simulink model "ATOM_simple_planning_simulator"  (R2026a)
settings: Solver=ode4  StopTime=50  FixedStep=0.01
StopFcn:
  | if exist('costmap_active','var') && ...
  |    exist('vehicle','var') && ...
  |    exist('parking_path','var') && ...
  |    ~isempty(parking_path)
  | 
  |     plotPlan(costmap_active, vehicle, parking_path);
  | else
  |     warning('No valid parking path is available for plotting.');
  | end
model workspace (MAT data in the model file):
  vehicle : object (value not decoded)
symbols that are objects in the model workspace (value not decoded): vehicle
undefined symbols (not defined in the file or in its folder): delta_f_LUT, gain4WS_LUT, k_ref_LUT, kappa_gain_BP, Ki, Kp, lateral, longitudinal, planning_validator, rr_gain_BP, rr_LUT, stanley, velocity_smoother
libraries: slpidlib x1, simulink x1
(part 6 of 7)

== matlab function ATOM_simple_planning_simulator/Subsystem/parkingNMPC ==
  settings: updateMethod=DISCRETE  sampleTime=0.04
  data: tx input; path_length output; ty input; tqz input; tqw input; tdf input; tdr input; tvx input; tax input; max_q output; X input; Y input; s_now output; ey_now output; qz input; qw input; vx input; ax_meas input; df input; dr input; x_now output; veh input; longitudinal_mode output; df_cmd output; dr_cmd output; nmpc_info output; segment_done output; segment_changed input; endpoint_error output; a_cmd_previous input; costmap input
function [path_length, max_q, s_now, ey_now, x_now, ...
    longitudinal_mode, df_cmd, dr_cmd, nmpc_info, ...
    segment_done, endpoint_error] = parkingNMPC( ...
    tx,ty,tqz,tqw,tdf,tdr,tvx,tax, ...
    X,Y,qz,qw,vx,ax_meas,df,dr,veh, ...
    segment_changed,a_cmd_previous,costmap)
persistent ref s_prev U_prev buf aBuf terminal_creep_steps

N  = 15;
nd = 6;

% Build the reference during the first execution.
if isempty(ref)
    ref = buildRef(tx,ty,tqz,tqw,tdf,tdr,tvx,tax);
end

if isempty(s_prev)
    s_prev = 0;
end

if isempty(U_prev)
    U_prev = repmat([df, dr], N, 1);
end

if isempty(buf)
    % Initialize the delayed-command history from the measured wheel angles.
    buf = repmat([df, dr], nd, 1);
end

% History of acceleration commands already sent to the vehicle.
% Three samples are retained because the acceleration delay is 0.10 s,
% equivalent to 2.5 controller intervals at Ts = 0.04 s.
if isempty(aBuf)
    aBuf = repmat(a_cmd_previous,3,1);
else
    aBuf = [aBuf(2:end); a_cmd_previous];
end

if isempty(terminal_creep_steps)
    terminal_creep_steps = 0.0;
end

% Rebuild the reference once when the segment changes.
if logical(segment_changed)
    ref = buildRef(tx,ty,tqz,tqw,tdf,tdr,tvx,tax);
    s_prev = 0;
    U_prev = repmat([df,dr],N,1);
    terminal_creep_steps = 0.0;
end
path_length = ref.s(end); max_q = max(ref.q);
[s_new, ey_now] = whereOnPath(ref, X, Y, s_prev);
s_now  = min(max(s_new, s_prev), s_prev + 0.5);   % never backwards, never a big jump forward
s_prev = s_now;

% --- the state of the car right now ---
psi   = 2*atan2(qz, qw);
x_now = [X; Y; psi; vx; df; dr; ax_meas]; %state of the nmpc controller
P     = carNumbers(veh);
M = mapNumbers(costmap);

% Remaining path distance used by the maneuver supervisor.
d_left = max(ref.s(end) - s_now, 0);

% The segment is complete only after reaching its end and stopping.
% Actual distance from the vehicle's rear axle to the segment endpoint.
endpoint_distance = hypot( ...
    X - ref.X(end), ...
    Y - ref.Y(end));

% Heading error relative to the segment endpoint, wrapped to [-pi, pi].
heading_difference = psi - ref.psi(end);

endpoint_heading_error = atan2( ...
    sin(heading_difference), ...
    cos(heading_difference));

% ---------------- Segment arrival and stop supervision ----------------
%
% Precise tolerance:
% Used to evaluate the final tracking quality.
%
% Arrival tolerance:
% Used to decide whether the stopped vehicle may proceed to the next
% forward/reverse segment.

end_distance_tolerance = 0.05;       % [m]
end_heading_tolerance  = 2*pi/180;   % [rad]

arrive_distance_tolerance = 0.20;       % [m]
arrive_heading_tolerance  = 5*pi/180;   % [rad]

stop_speed_tolerance = 0.02;         % [m/s]

% Because s_now is not allowed to decrease, end_reached remains true
% after the vehicle reaches the final path progress.
end_reached = ...
    d_left <= 0.02;

% High-accuracy endpoint condition.
pose_acceptable = ...
    (endpoint_distance <= end_distance_tolerance) && ...
    (abs(endpoint_heading_error) <= end_heading_tolerance);

% Practical condition for authorizing the next gear segment.
pose_arrived = ...
    (endpoint_distance <= arrive_distance_tolerance) && ...
    (abs(endpoint_heading_error) <= arrive_heading_tolerance);

% The vehicle must be nearly stationary before changing segments.
stopped = ...
    abs(vx) <= stop_speed_tolerance;

% Advance to the next segment only after reaching the endpoint progress,
% stopping, and satisfying the practical arrival tolerance.
segment_done = ...
    end_reached && ...
    stopped && ...
    pose_arrived;

% If the vehicle stops outside the arrival tolerance, keep the current
% segment active and report the failure through the controller status.
arrival_failed = ...
    end_reached && ...
    stopped && ...
    ~pose_arrived;

% Permanent endpoint diagnostics:
%   element 1: position error [m]
%   element 2: signed heading error [deg]
endpoint_error = [ ...
    endpoint_distance; ...
    endpoint_heading_error*180/pi];

% Longitudinal modes:
%   0 = follow the planned velocity profile
%   2 = stop
%
% Once endpoint progress is reached, stop mode remains active.
% Terminal creep mode is deliberately removed.
longitudinal_mode = 0.0;

if end_reached
    longitudinal_mode = 2.0;
end

% --- steering ---
use_nmpc = true;      % false = D1 baseline (follow the plan blindly)
w = [10 10 1 0.1];     % weights: side error, heading error, wheel error, command jumps

if use_nmpc
    x0   = x_now;                                          % start from the real car
    cost = @(u) score( ...
        reshape(u,N,2), ...
        x0, ...
        s_now, ...
        buf, ...
        aBuf, ...
        ref, ...
        P, ...
        w, ...
        longitudinal_mode);

    nonlinear_constraint = @(u) collisionConstraints( ...
        u, ...
        x0, ...
        s_now, ...
        buf, ...
        aBuf, ...
        ref, ...
        P, ...
        M, ...
        longitudinal_mode);

    lb   = -P.steerMax*ones(2*N,1);                        % wheel limits
    ub   =  P.steerMax*ones(2*N,1);
    % Shared tolerance for the optimizer and the independent collision check.
    collision_tolerance = 1e-6;
    
    opts = optimoptions('fmincon', ...
        'Algorithm', 'sqp', ...
        'Display', 'none', ...
        'MaxIterations', 30, ...
        'ConstraintTolerance', collision_tolerance);
    solve_start = tic;
    
    % Optimize the front and rear steering commands.
    % Steering-angle limits are hard constraints.
    % Command changes are discouraged by the dU term in the cost function.
    [u, J_best, flag, solver_output] = fmincon( ...
        cost, U_prev(:), ...
        [], [], [], [], ...
        lb, ub, ...
        nonlinear_constraint, opts);
    
    solve_time = toc(solve_start);
    % Check whether the returned cost and commands are finite.
    finite_solution = ...
        isfinite(J_best) && ...
        all(isfinite(u));

    % Small tolerance for numerical round-off at the steering limits.
    bound_tolerance = 1e-9;

    % Check whether all optimized commands respect their bounds.
    inside_bounds = ...
        all(u >= lb - bound_tolerance) && ...
        all(u <= ub + bound_tolerance);

    % Verify the nonlinear collision constraints independently after
    % fmincon returns its candidate solution.
    collision_feasible = false;

    % Do not evaluate geometric constraints using nonfinite commands or
    % a candidate already declared invalid by the solver.
    if finite_solution && flag >= 0

        [candidate_collision_constraints,~] = ...
            collisionConstraints( ...
            u, ...
            x0, ...
            s_now, ...
            buf, ...
            aBuf, ...
            ref, ...
            P, ...
            M, ...
            longitudinal_mode);

        collision_feasible = ...
            all(isfinite(candidate_collision_constraints)) && ...
            all(candidate_collision_constraints <= ...
            collision_tolerance);
    end


    % Classify the optimization result.
    if ~finite_solution || ...
       ~inside_bounds || ...
       ~collision_feasible || ...
       flag < 0

        % The optimizer returned an unusable result.
        controller_status = 2;

    elseif flag == 0 || solve_time > P.Ts

        % The result is usable, but the solver did not converge normally
        % or exceeded the controller sampling period.
        controller_status = 1;

    else

        % The solver returned a normal valid result.
        controller_status = 0;

    end

    % Endpoint-arrival diagnostics.
    % Preserve status 2 when the optimizer result itself is invalid.
    %
    % Status 5:
    %   stopped outside the 0.20 m / 5 degree arrival tolerance.
    %
    % Status 4:
    %   segment accepted using the arrival tolerance, but outside the
    %   more precise 0.05 m / 2 degree quality tolerance.
    
    if controller_status ~= 2
    
        if arrival_failed
            controller_status = 5;
    
        elseif segment_done && ~pose_acceptable
            controller_status = 4;
        end
    
    end
        
    % If the new optimizer result is unusable, verify whether the
    % remaining previous steering plan is still safe from the current
    % measured state and with the current costmap.
    fallback_collision_feasible = false;

    if controller_status == 2

        fallback_u = U_prev(:);

        fallback_finite = ...
            all(isfinite(fallback_u));

        fallback_inside_bounds = ...
            all(fallback_u >= lb - bound_tolerance) && ...
            all(fallback_u <= ub + bound_tolerance);

        if fallback_finite && fallback_inside_bounds

            [fallback_collision_constraints,~] = ...
                collisionConstraints( ...
                fallback_u, ...
                x0, ...
                s_now, ...
                buf, ...
                aBuf, ...
                ref, ...
                P, ...
                M, ...
                longitudinal_mode);

            fallback_collision_feasible = ...
                all(isfinite(fallback_collision_constraints)) && ...
                all(fallback_collision_constraints <= ...
                collision_tolerance);
        end
    end

    % Convert the new optimizer result into an N-by-2 steering plan.
    U_candidate = reshape(u, N, 2);
    
    % Select the steering plan that the controller is allowed to use.
    if controller_status == 2

        if fallback_collision_feasible

            % The new result is unusable, but the remaining previous
            % plan is still collision-free from the current state.
            U_selected = U_prev;

        else

            % Neither the new solution nor the previous plan is safe.
            % Request braking from the separate longitudinal controller.
            longitudinal_mode = 2.0;

            % Hold the current measured steering angles while stopping.
            hold_front = max( ...
                -P.steerMax, ...
                min(P.steerMax,df));

            hold_rear = max( ...
                -P.steerMax, ...
                min(P.steerMax,dr));

            U_selected = repmat( ...
                [hold_front,hold_rear], ...
                N,1);

            % Status 6 means emergency stop caused by the absence of a
            % collision-feasible steering sequence.
            controller_status = 6;
        end

    else
    
        % Status 0: normal solution.
        % Status 1: degraded but numerically valid solution.
        U_selected = U_candidate;
    
    end
    
    % Send only the first command from the selected plan.
    df_cmd = U_selected(1,1);
    dr_cmd = U_selected(1,2);
    
    % Add the command that was actually sent to the steering-delay queue.
    buf = [buf(2:end,:); U_selected(1,:)];
    
    % Prepare the remaining selected plan as the next warm start.
    U_prev = [U_selected(2:end,:); U_selected(end,:)];
    nmpc_info = [ ...
        double(J_best); ...
        double(flag); ...
        double(solve_time); ...
        double(solver_output.iterations); ...
        double(solver_output.funcCount); ...
        double(controller_status)];
else
    df_cmd = lookupS(ref.s, ref.df, s_now);
    dr_cmd = lookupS(ref.s, ref.dr, s_now);
    nmpc_info = [0; 0; 0; 0; 0; 3];
end
end

%--------------------------------------------------------------------------
function P = carNumbers(veh)
% All fields must be created before the structure is read.

collisionMargin = 0.5;

P.L        = veh(3);
P.steerMax = veh(10);
P.aMax     = veh(16);
P.rateLim  = veh(18);
P.tau      = veh(22);
P.vMax     = 2.0;
P.Ts       = 0.04;
P.accDelay = veh(19);
P.accTau   = veh(20);
P.aCmdMax  = 1.0;

P.footprintMargin = collisionMargin;

P.footprintBack = ...
    -(veh(6) + collisionMargin/2);

P.footprintFront = ...
    veh(3) + veh(5) + collisionMargin/2;

P.footprintHalfWidth = ...
    (veh(4) + veh(7) + veh(8) + collisionMargin)/2;
end

%--------------------------------------------------------------------------
function M = mapNumbers(costmap)

resolution = double(costmap.info.resolution);

M.res = resolution;
M.width = double(costmap.info.width);
M.height = double(costmap.info.height);

M.originX = double(costmap.info.origin.position.x);
M.originY = double(costmap.info.origin.position.y);

M.grid = double(costmap.data)/100;

M.cellHalf = resolution/2;
end

%--------------------------------------------------------------------------
function [x1,aBuf1] = predictStep( ...
    x0,aBuf,aCmd,dfc,drc,P)
% Predict the vehicle over one 0.04 s controller interval.

X   = x0(1);
Y   = x0(2);
psi = x0(3);
vx  = x0(4);
df  = x0(5);
dr  = x0(6);
ax  = x0(7);

%% Steering actuator

ddf = max( ...
    -P.rateLim, ...
    min(P.rateLim,(dfc-df)/P.tau));

ddr = max( ...
    -P.rateLim, ...
    min(P.rateLim,(drc-dr)/P.tau));

df1 = max( ...
    -P.steerMax, ...
    min(P.steerMax,df+P.Ts*ddf));

dr1 = max( ...
    -P.steerMax, ...
    min(P.steerMax,dr+P.Ts*ddr));

%% Acceleration delay and actuator lag

% The 0.04 s interval is divided into two 0.02 s parts.
h = 0.5*P.Ts;

% For a 0.10 s transport delay, the delayed command changes halfway
% through the current 0.04 s interval.
aDelayedFirst  = aBuf(1);
aDelayedSecond = aBuf(2);

% First half of the acceleration-actuator response.
axHalf = ax + ...
    h*(aDelayedFirst-ax)/P.accTau;

axHalf = max( ...
    -P.aMax, ...
    min(P.aMax,axHalf));

% Second half of the acceleration-actuator response.
ax1 = axHalf + ...
    h*(aDelayedSecond-axHalf)/P.accTau;

ax1 = max( ...
    -P.aMax, ...
    min(P.aMax,ax1));

% Integrate acceleration over the two half-steps.
deltaVFirst = ...
    0.5*h*(ax+axHalf);

deltaVSecond = ...
    0.5*h*(axHalf+ax1);

vx1 = vx + deltaVFirst + deltaVSecond;

vx1 = max( ...
    -P.vMax, ...
    min(P.vMax,vx1));

% Store the acceleration command predicted for the current cycle.
aBuf1 = [aBuf(2:end); aCmd];

%% Vehicle motion

drMid = 0.5*(dr+dr1);
vxMid = 0.5*(vx+vx1);

dRear = ...
    vxMid*P.Ts/max(cos(drMid),0.1);

[X1,Y1,psi1] = bicycleGetPose( ...
    X,Y,psi,df1,dr1,P.L,dRear);

x1 = [X1;Y1;psi1;vx1;df1;dr1;ax1];

end

%--------------------------------------------------------------------------
function J = score( ...
    U,x0,s0,buf,aBuf,ref,P,w,longitudinal_mode)
Ucmd = [buf; U];

x = x0;
s = s0;
J = 0;

% Each objective evaluation must start from the same real acceleration
% command history. Only this local copy will be changed during prediction.
aBufPrediction = aBuf;

% Start from the maneuver-supervisor mode active in the real system.
modePrediction = longitudinal_mode;
% How bad is this imagined future? Lower is better.
Ucmd = [buf; U];                  % the queue plays first, then the new plan
x = x0;  s = s0;  J = 0;
for k = 1:size(Ucmd,1)

    % The longitudinal controller is separate from the steering NMPC.
    % The steering prediction therefore uses the planned feedforward
    % acceleration as a known external input.
    % Once predicted endpoint progress is reached, remain in stop mode.
    dLeftPrediction = max(ref.s(end)-s,0.0);
    
    if dLeftPrediction <= 0.02
        modePrediction = 2.0;
    end
    
    % Predict what the separate longitudinal controller will command.
    aCmdPrediction = longitudinalCommandPrediction( ...
        ref, ...
        s, ...
        x(4), ...
        modePrediction, ...
        P);
    
    % Predict acceleration actuator, speed, steering and vehicle motion.
    [x,aBufPrediction] = predictStep( ...
        x, ...
        aBufPrediction, ...
        aCmdPrediction, ...
        Ucmd(k,1), ...
        Ucmd(k,2), ...
        P);

    [s,ey] = whereOnPath(ref,x(1),x(2),s);
    dpsi = x(3) - lookupS(ref.s, ref.psi, s);
    epsi = atan2(sin(dpsi), cos(dpsi));
    edf  = x(5) - lookupS(ref.s, ref.df, s);
    edr  = x(6) - lookupS(ref.s, ref.dr, s);
    J = J + w(1)*ey^2 + w(2)*epsi^2 + w(3)*(edf^2 + edr^2);
end
dU = diff([buf(end,:); U]);       % jumps between consecutive commands
J  = J + w(4)*sum(dU(:).^2);
end

%--------------------------------------------------------------------------
function a_cmd = longitudinalCommandPrediction( ...
    ref, s, vx, longitudinal_mode, P)
% Predict the acceleration command that the separate longitudinal
% controller will generate.

Kp = 1.0;
Kp_stop = 5.0;
terminal_creep_speed = 0.05;

v_ref = lookupS(ref.s,ref.v,s);
a_ref = lookupS(ref.s,ref.a,s);

gear = ref.gear;
Kp_active = Kp;

if longitudinal_mode == 2.0

    % Stop mode.
    v_ref = 0.0;
    a_ref = 0.0;
    Kp_active = Kp_stop;

elseif longitudinal_mode == 1.0

    % Terminal-creep mode.
    v_ref = gear*terminal_creep_speed;
    a_ref = 0.0;

end

speed_error = v_ref-vx;

speed_in_gear = gear*vx;
reference_speed_in_gear = gear*v_ref;
feedforward_in_gear = gear*a_ref;

a_feedforward = a_ref;

% Apply braking feedforward only while the vehicle is moving faster
% than its reference in the intended gear direction.
if feedforward_in_gear < 0.0 && ...
        speed_in_gear <= reference_speed_in_gear

    a_feedforward = 0.0;

end

a_unsaturated = ...
    a_feedforward + Kp_active*speed_error;

a_cmd = max( ...
    -P.aCmdMax, ...
    min(P.aCmdMax,a_unsaturated));

end

%--------------------------------------------------------------------------
function v = lookupS(sv, vv, s)
% Value of vv at distance s along the route (straight line between points).
n = numel(sv);
v = vv(n);
if s <= sv(1), v = vv(1); return; end
if s >= sv(n), return; end
for i = 1:n-1
    if s <= sv(i+1)
        ds = sv(i+1) - sv(i);
        if ds < 1e-12
            v = vv(i+1);
        else
            v = vv(i) + (s - sv(i))/ds*(vv(i+1) - vv(i));
        end
        return;
    end
end
end

%--------------------------------------------------------------------------
function ref = buildRef(tx, ty, tqz, tqw, tdf, tdr, tvx, tax)
% The route, labelled by how many metres along it each point is.
n = numel(tx);

psi = 2*atan2(tqz(:), tqw(:));
for i = 2:n
    d = psi(i) - psi(i-1);
    psi(i) = psi(i) - 2*pi*round(d/(2*pi));
end

s = zeros(n,1);
for i = 2:n
    s(i) = s(i-1) + hypot(tx(i)-tx(i-1), ty(i)-ty(i-1));
end

q = zeros(n,1);
for i = 1:n-1
    ds   = max(s(i+1) - s(i), 1e-9);
    q(i) = max(abs(tdf(i+1)-tdf(i)), abs(tdr(i+1)-tdr(i))) / ds;
end
q(n) = q(n-1);

ref.X  = tx(:);   ref.Y  = ty(:);   ref.psi = psi;
ref.df = tdf(:);  ref.dr = tdr(:);
ref.s  = s;       ref.q  = q;
ref.v = tvx(:);
ref.a = tax(:);

% Direction of this trajectory segment:
% +1 means forward, -1 means reverse.
% Direction of this trajectory segment:
% +1 means forward, -1 means reverse.
% The first velocity can be zero because every smoothed segment starts
% from rest, so search for the first nonzero velocity value.
gear = 1;

for k = 1:numel(tvx)
    if abs(tvx(k)) > 1e-6
        gear = sign(tvx(k));
        break;
    end
end

ref.gear = gear;
end

%--------------------------------------------------------------------------
function [s, ey] = whereOnPath(ref, X, Y, s_guess)
% Closest point on the route to (X,Y).
%   s  : how far along the route that point is
%   ey : how far to the side the car is (left positive)
n = numel(ref.s);
best = inf;  s = s_guess;  ey = 0;
win  = 1.5;

for pass = 1:2
    for i = 1:n-1
        if abs(ref.s(i) - s_guess) > win
            continue;
        end
        ax = ref.X(i);   ay = ref.Y(i);
        bx = ref.X(i+1); by = ref.Y(i+1);
        L2 = (bx-ax)^2 + (by-ay)^2;
        t  = ((X-ax)*(bx-ax) + (Y-ay)*(by-ay)) / max(L2, 1e-12);
        t  = min(max(t, 0), 1);
        px = ax + t*(bx-ax);   py = ay + t*(by-ay);
        d2 = (X-px)^2 + (Y-py)^2;
        if d2 < best
            best = d2;
            s  = ref.s(i) + t*(ref.s(i+1) - ref.s(i));
            ey = sign((bx-ax)*(Y-ay) - (by-ay)*(X-ax)) * sqrt(d2);
        end
    end
    if best < inf, break; end
    win = inf;
end
end

%--------------------------------------------------------------------------
function cPose = poseCollisionConstraint(X,Y,psi,P,M) %This function is added in our way for the implementation of the non-linear hard constraint of the obstacle avoidance
% Continuous collision measure for one predicted vehicle pose.
%
% fmincon convention:
%   cPose < 0  : collision-free
%   cPose = 0  : touching the obstacle or map boundary
%   cPose > 0  : collision or map-boundary violation

% Nearby obstacles begin influencing the constraint from this distance.
% This is not an additional vehicle safety margin.
influenceDistance = 1.0;

% Prevent exact geometric touching from being accepted because of
% numerical round-off.
numericalClearance = 1e-4;

ct = cos(psi);
st = sin(psi);

%% Enlarged vehicle rectangle

back = P.footprintBack;
front = P.footprintFront;
halfWidth = P.footprintHalfWidth;

vehicleCentreOffset = 0.5*(front + back);
vehicleHalfLength = 0.5*(front - back);

vehicleCentreX = X + ct*vehicleCentreOffset;
vehicleCentreY = Y + st*vehicleCentreOffset;

% Projection of the rotated vehicle rectangle onto the world axes.
vehicleProjectionX = ...
    vehicleHalfLength*abs(ct) + halfWidth*abs(st);

vehicleProjectionY = ...
    vehicleHalfLength*abs(st) + halfWidth*abs(ct);

vehicleMinX = vehicleCentreX - vehicleProjectionX;
vehicleMaxX = vehicleCentreX + vehicleProjectionX;
vehicleMinY = vehicleCentreY - vehicleProjectionY;
vehicleMaxY = vehicleCentreY + vehicleProjectionY;

%% Map-boundary constraint

mapMinX = M.originX - M.cellHalf;
mapMaxX = M.originX + (M.width-1)*M.res + M.cellHalf;

mapMinY = M.originY - M.cellHalf;
mapMaxY = M.originY + (M.height-1)*M.res + M.cellHalf;

boundaryConstraint = max( ...
    max( ...
        mapMinX - vehicleMinX, ...
        vehicleMaxX - mapMaxX), ...
    max( ...
        mapMinY - vehicleMinY, ...
        vehicleMaxY - mapMaxY));

%% Find nearby costmap cells

searchHalfX = ...
    vehicleProjectionX + M.cellHalf + influenceDistance;

searchHalfY = ...
    vehicleProjectionY + M.cellHalf + influenceDistance;

ix0 = ceil( ...
    (vehicleCentreX-searchHalfX-M.originX)/M.res);

ix1 = floor( ...
    (vehicleCentreX+searchHalfX-M.originX)/M.res);

iy0 = ceil( ...
    (vehicleCentreY-searchHalfY-M.originY)/M.res);

iy1 = floor( ...
    (vehicleCentreY+searchHalfY-M.originY)/M.res);

ix0 = max(0,ix0);
ix1 = min(M.width-1,ix1);

iy0 = max(0,iy0);
iy1 = min(M.height-1,iy1);

% A value of -influenceDistance is safely feasible.
obstacleConstraint = -influenceDistance;

% Projection of a square costmap cell onto either vehicle axis.
cellProjectionRotated = ...
    M.cellHalf*(abs(ct) + abs(st));

%% Rectangle-versus-cell constraints

if ix0 <= ix1 && iy0 <= iy1

    for iy = iy0:iy1
        for ix = ix0:ix1

            cellValue = M.grid(iy+1,ix+1);

            % Occupied cells are >= 1.
            % Unknown cells are negative and are also unsafe.
            if cellValue >= 1.0 || cellValue < 0.0

                cellX = M.originX + ix*M.res;
                cellY = M.originY + iy*M.res;

                dx = cellX - vehicleCentreX;
                dy = cellY - vehicleCentreY;

                % Overlap on the two world axes.
                overlapWorldX = ...
                    vehicleProjectionX + M.cellHalf - abs(dx);

                overlapWorldY = ...
                    vehicleProjectionY + M.cellHalf - abs(dy);

                % Cell position expressed along the vehicle axes.
                distanceLongitudinal = ct*dx + st*dy;
                distanceLateral = -st*dx + ct*dy;

                % Overlap on the two vehicle axes.
                overlapLongitudinal = ...
                    vehicleHalfLength + ...
                    cellProjectionRotated - ...
                    abs(distanceLongitudinal);

                overlapLateral = ...
                    halfWidth + ...
                    cellProjectionRotated - ...
                    abs(distanceLateral);

                % SAT collision measure for this occupied cell.
                cellConstraint = min( ...
                    min(overlapWorldX,overlapWorldY), ...
                    min(overlapLongitudinal,overlapLateral));

                obstacleConstraint = max( ...
                    obstacleConstraint, ...
                    cellConstraint);
            end
        end
    end
end

% The worst condition determines whether this pose is feasible.
cPose = ...
    max(boundaryConstraint,obstacleConstraint) + ...
    numericalClearance;
end

%--------------------------------------------------------------------------
function [c,ceq] = collisionConstraints( ...
    u,x0,s0,buf,aBuf,ref,P,M,longitudinal_mode)%This function is added in our way for the implementation of the non-linear hard constraint of the obstacle avoidance
% Evaluate obstacle constraints across the complete predicted motion.
%
% u:
%   30-by-1 optimization vector containing 15 front commands followed
%   by 15 rear commands.
%
% c:
%   One inequality value for every predicted pose.
%   fmincon will eventually require every element of c to satisfy:
%
%       c(k) <= 0
%
% ceq:
%   Empty because this NMPC has no nonlinear equality constraints.

N = 15;

% Convert the solver vector into:
%
%       row k = [front command, rear command]
%
U = reshape(u,N,2);

% The six commands already waiting in the steering transport-delay
% queue act first. The fifteen candidate commands act afterward.
Ucmd = [buf; U];

numberOfPredictedSteps = size(Ucmd,1);

% Six queued steps plus fifteen candidate steps gives 21 constraints.
c = zeros(numberOfPredictedSteps,1);

% No nonlinear equality constraints.
ceq = zeros(0,1);

% Every solver evaluation starts from the current measured state.
x = x0;
s = s0;

% Use local prediction copies. Persistent real-controller data is
% therefore not changed while fmincon tests candidate sequences.
aBufPrediction = aBuf;
modePrediction = longitudinal_mode;

for k = 1:numberOfPredictedSteps

    %% Reproduce the longitudinal prediction used by score()

    dLeftPrediction = max(ref.s(end)-s,0.0);

    if dLeftPrediction <= 0.02
        modePrediction = 2.0;
    end

    aCmdPrediction = longitudinalCommandPrediction( ...
        ref, ...
        s, ...
        x(4), ...
        modePrediction, ...
        P);

    %% Predict the next complete vehicle state

    [x,aBufPrediction] = predictStep( ...
        x, ...
        aBufPrediction, ...
        aCmdPrediction, ...
        Ucmd(k,1), ...
        Ucmd(k,2), ...
        P);

    %% Update predicted progress along the reference path

    [s,~] = whereOnPath( ...
        ref, ...
        x(1), ...
        x(2), ...
        s);

    %% Evaluate the predicted footprint against the costmap

    c(k) = poseCollisionConstraint( ...
        x(1), ...
        x(2), ...
        x(3), ...
        P, ...
        M);
end
end

== matlab function ATOM_simple_planning_simulator/Vehicle_Model/Vehicle Dynamics/MATLAB Function ==
  data: state input Bus: VehicleInternalStateBus size=1; d_state output Bus: VehicleInternalStateBus size=1; command input Bus: ControlCMDBus size=1; veh input; rear_steering_command input
function d_state = vehicleDynamics(state, command, veh, rear_steering_command)

%%%%%%%%%%%%%%%%%%%%%%%%%%%%%%%%%%%%%%
%%%%%%%%%%%%%%%%%%%%%%%%%%%%%%%%%%%%%%
% Description:
% This vehicleDynamics model follows DELAY_STEER_ACC_GEARED
% model, it doesn't presents a model for gear management
% since its not something we're going to modify on Autoware for 4WS
% implementation.
%
% Inputs:
% - state: VehicleInternalStateBus. It contains the state of the vehicle
%          at time instant t. 
% - command: /control/command/control_cmd topic --> ControlCMDBus.
%          It contains the desired acc and steering commands coming from
%          the control region.
%
% - Parameters
% - vehicle: vehicle parameters struct defined in vehicleParameters.m.

% Outputs: 
% - d_state: It contains the derivative of the state of the vehicle at time
%          instant t+1.
%%%%%%%%%%%%%%%%%%%%%%%%%%%%%%%%%%%%%%
%%%%%%%%%%%%%%%%%%%%%%%%%%%%%%%%%%%%%%


% inside MATLAB Function: input is veh_in (1xN double)
v = veh; % 1xN numeric row

vehicle.param.wheel_radius    = v(1);
vehicle.param.wheel_width     = v(2);
vehicle.param.wheel_base      = v(3);
vehicle.param.wheel_tread     = v(4);
vehicle.param.front_overhang  = v(5);
vehicle.param.rear_overhang   = v(6);
vehicle.param.left_overhang   = v(7);
vehicle.param.right_overhang  = v(8);
vehicle.param.vehicle_height  = v(9);
vehicle.param.max_steer_angle = v(10);

% decode integer-coded enums (example)
vehicle.sim.vehicle_model_type = int32(v(11));    % or map to strings if needed
vehicle.sim.initialize_source  = int32(v(12));

vehicle.sim.timer_sampling_time_ms = v(13);
vehicle.sim.add_measurement_noise = logical(v(14));
vehicle.sim.vel_lim        = v(15);
vehicle.sim.vel_rate_lim   = v(16);
vehicle.sim.steer_lim      = v(17);
vehicle.sim.steer_rate_lim = v(18);
vehicle.sim.acc_time_delay = v(19);
vehicle.sim.acc_time_constant = v(20);
vehicle.sim.steer_time_delay   = v(21);
vehicle.sim.steer_time_constant= v(22);
vehicle.sim.x_stddev = v(23);
vehicle.sim.y_stddev = v(24);
vehicle.sim.steer_dead_band = v(25);
vehicle.sim.steer_bias = v(26);
vehicle.sim.debug_acc_scaling_factor = v(27);
vehicle.sim.debug_steer_scaling_factor = v(28);

% Parameter for 4WS
vehicle.param.rear_steering_ratio = veh(29);
rear_steering_ratio = vehicle.param.rear_steering_ratio;

%% ==========================
% Saturation function
% ===========================

sat = @(val, upper, lower) min(max(val,lower),upper);



%% ==========================
% Current state
% ===========================

vx = sat( ...
    state.vx,...
    vehicle.sim.vel_lim,...
   -vehicle.sim.vel_lim);


acc = sat( ...
    state.acc,...
    vehicle.sim.vel_rate_lim,...
   -vehicle.sim.vel_rate_lim);


yaw = state.yaw;

steer_front = state.steer_front;
steer_rear = state.steer_rear;          % Modified for 4WS  


%% ==========================
% Input commands
% ===========================

acc_des = sat( ...
    command.longitudinal.acceleration,...
    vehicle.sim.vel_rate_lim,...
   -vehicle.sim.vel_rate_lim);


acc_des = acc_des * ...
    vehicle.sim.debug_acc_scaling_factor;



steer_front_des = sat( ...
    command.lateral.steering_tire_angle,...
    vehicle.sim.steer_lim,...
   -vehicle.sim.steer_lim);


steer_front_des = steer_front_des * ...
    vehicle.sim.debug_steer_scaling_factor;

steer_rear_des = sat( ...                                            % Modified for 4WS
    rear_steering_command,...
    vehicle.sim.steer_lim,...
    -vehicle.sim.steer_lim);


steer_rear_des = steer_rear_des * ...                                % Modified for 4WS
    vehicle.sim.debug_steer_scaling_factor;



%% ==========================
% Steering dynamics
% ===========================

% getSteer() in simple_planning_simulator corresponds to state.steer
% From the phisical vehicle front_steer and rear_steer are measured.

steer_diff_front = steer_front - steer_front_des;

steer_diff_rear = steer_rear  - steer_rear_des;             % Modified for 4WS


% dead band

if steer_diff_front > vehicle.sim.steer_dead_band

    steer_diff_with_dead_band_front = ...
        steer_diff_front - vehicle.sim.steer_dead_band;


elseif steer_diff_front < -vehicle.sim.steer_dead_band

    steer_diff_with_dead_band_front = ...
        steer_diff_front + vehicle.sim.steer_dead_band;


else

    steer_diff_with_dead_band_front = 0;

end



if steer_diff_rear > vehicle.sim.steer_dead_band            % Modified for 4WS

    steer_diff_with_dead_band_rear = ...
        steer_diff_rear - vehicle.sim.steer_dead_band;


elseif steer_diff_rear < -vehicle.sim.steer_dead_band

    steer_diff_with_dead_band_rear = ...
        steer_diff_rear + vehicle.sim.steer_dead_band;


else

    steer_diff_with_dead_band_rear = 0;

end



steer_rate_front = sat( ...
    -steer_diff_with_dead_band_front / vehicle.sim.steer_time_constant,...
     vehicle.sim.steer_rate_lim,...
    -vehicle.sim.steer_rate_lim);

steer_rate_rear = sat( ...                                                  % Modified for 4WS
    -steer_diff_with_dead_band_rear / vehicle.sim.steer_time_constant,...
    vehicle.sim.steer_rate_lim,...
    -vehicle.sim.steer_rate_lim);



%% ==========================
% State derivative
% ===========================

%--------------------------------------------------------------
% 4WS kinematic bicycle model
%
% Assumptions:
%   - Pure rolling
%   - alpha_f = alpha_r = 0
%   - No tire dynamics
%   - No lateral slip dynamics
%
% beta is the geometric vehicle sideslip angle. Since Autoware defines
% reference frame of the vehicle equal to centre of the rear axle, then
% beta = steer_rear
%--------------------------------------------------------------

L = vehicle.param.wheel_base;


beta = steer_rear;                              % Modified for 4WS


vel = vx/cos(beta);                             % Modified for 4WS


yaw_rate = ...                                  % Modified for 4WS
    (vx/L) * ...
    (tan(steer_front)-tan(steer_rear));


d_state.x = vel*cos(yaw + beta);                % Modified for 4WS

d_state.y = vel*sin(yaw + beta);                % Modified for 4WS


d_state.yaw = yaw_rate;                         % Modified for 4WS


d_state.vx = acc + yaw_rate*vel*sin(beta);


d_state.steer_front = steer_rate_front;

d_state.steer_rear = steer_rate_rear;           % Modified for 4WS

d_state.acc = ...
    -(acc-acc_des)/vehicle.sim.acc_time_constant;

end

== matlab function ATOM_simple_planning_simulator/Vehicle_Model/localization//acceleration function ==
  data: state input Bus: VehicleInternalStateBus; accel output Bus: AccelerationBus; veh input
function accel = IntStateToAccelerationState(state,veh)

L = veh(3);

vx = state.vx;
ax = state.acc;

delta_f = state.steer_front;
delta_r = state.steer_rear;

yaw_rate = (vx/L)*(tan(delta_f)-tan(delta_r));

ay = vx*yaw_rate;

accel.acceleration.linear.x = ax;
accel.acceleration.linear.y = ay;
accel.acceleration.linear.z = 0;

accel.acceleration.angular.x = 0;
accel.acceleration.angular.y = 0;
accel.acceleration.angular.z = 0;

end

== matlab function ATOM_simple_planning_simulator/Vehicle_Model/localization//kinematic_state function ==
  data: state input Bus: VehicleInternalStateBus; kinematic output Bus: KinematicStateBus; veh input
function kinematic = IntStateToKinematicState(state, veh)


%% Vehicle parameters

L = veh(3);


%% Current state

x = state.x;
y = state.y;
yaw = state.yaw;



% NOTE:
% vx is the longitudinal velocity expressed in the vehicle body frame
% (base_link located at the center of the rear axle).
% The vehicle speed magnitude is reconstructed as
%
%   v = vx / cos(delta_r)
%
% under the pure-rolling assumption (alpha_f = alpha_r = 0).

vx = state.vx;

steer_front = state.steer_front;
steer_rear  = state.steer_rear;


%% Pose

kinematic.pose.position.x = x;
kinematic.pose.position.y = y;
kinematic.pose.position.z = 0;


[qx,qy,qz,qw] = yawToQuaternion(yaw);

% quaternion from yaw only

kinematic.pose.orientation.x = qx;
kinematic.pose.orientation.y = qy;
kinematic.pose.orientation.z = qz;
kinematic.pose.orientation.w = qw;



%% Twist

% Body frame velocity

kinematic.twist.linear.x = vx;

kinematic.twist.linear.y = ...              % Modified for 4WS considering beta = steer_rear
    vx*tan(steer_rear);

kinematic.twist.linear.z = 0;



% Angular velocity

kinematic.twist.angular.x = 0;
kinematic.twist.angular.y = 0;

kinematic.twist.angular.z = ...
    (vx/L) * ...
    (tan(steer_front)-tan(steer_rear));


end

== matlab function ATOM_simple_planning_simulator/Plot vehicle1/Plot Vehicle Rear reference frame ==
  settings: updateMethod=DISCRETE
  data: kinematic input Bus: KinematicStateBus; steer_front input double; steer_rear input double; veh input; traj input; costmap input
   function plotVehicleRear(kinematic, steer_front, steer_rear, veh, traj, costmap)
  coder.extrinsic('imagesc','colormap','evalin');
%% Vehicle parameters

L  = veh(3);
track = veh(4);

front_overhang = veh(5);
rear_overhang  = veh(6);
left_overhang = veh(7);
right_overhang = veh(8);

vehicle_length  = L + front_overhang + rear_overhang;
vehicle_width = track + left_overhang + right_overhang;

wheel_width = veh(2);
wheel_radius = veh(1);

%% Reference trajectory

x_ref = evalin('base', 'parking_path(:,1)');
y_ref = evalin('base', 'parking_path(:,2)');


%% Current kinematic state

x = kinematic.pose.position.x;
y = kinematic.pose.position.y;

qz = kinematic.pose.orientation.z;
qw = kinematic.pose.orientation.w;

yaw = 2*atan2(qz,qw);

vx = kinematic.twist.linear.x;

steer_front = steer_front;
steer_rear = steer_rear;

%% Position and orientation vehicle body

vehicle_body = [L+front_overhang vehicle_width/2;
                L+front_overhang -vehicle_width/2;
                -rear_overhang -vehicle_width/2;
                -rear_overhang vehicle_width/2;
                L+front_overhang vehicle_width/2];

R_body = [ cos(yaw) -sin(yaw)
    sin(yaw)  cos(yaw) ];

body_world = (R_body*vehicle_body')';

body_world(:,1)=body_world(:,1)+x;
body_world(:,2)=body_world(:,2)+y;


%% Position and orientation wheels

wheel_body = [wheel_radius  wheel_width/2
                wheel_radius -wheel_width/2
                -wheel_radius -wheel_width/2
                -wheel_radius  wheel_width/2
                wheel_radius  wheel_width/2];

FL = [L  track/2];
FR = [L -track/2];
RL = [0  track/2];
RR = [0 -track/2];

centers = [FL;
    FR;
    RL;
    RR];

centers = (R_body*centers')';

centers(:,1) = centers(:,1)+x;
centers(:,2) = centers(:,2)+y;

wheelFL = transformWheel(centers(1,:),steer_front,yaw,wheel_body);
wheelFR = transformWheel(centers(2,:),steer_front,yaw,wheel_body);
wheelRL = transformWheel(centers(3,:),steer_rear,yaw,wheel_body);
wheelRR = transformWheel(centers(4,:),steer_rear,yaw,wheel_body);



persistent hFig
persistent ax
persistent hBody
persistent hWheelFL
persistent hWheelFR
persistent hWheelRL
persistent hWheelRR
persistent hTrajectory
persistent TrajX
persistent TrajY
persistent hRefTraj 


if isempty(hBody)
    hFig = figure(20);
    clf

    ax = axes(hFig);

    hold(ax,'on')
    axis(ax,'equal')
    grid(ax,'on')


    xlabel(ax,'x [m]')
    ylabel(ax,'y [m]')

    % --- obstacles: the same costmap the planner used ---
    res = double(costmap.info.resolution);
    W   = double(costmap.info.width);
    H   = double(costmap.info.height);
    ox  = double(costmap.info.origin.position.x);
    oy  = double(costmap.info.origin.position.y);
    g   = double(costmap.data);
    imagesc(ax, ox+(0:W-1)*res, oy+(0:H-1)*res, g, 'AlphaData', (g>=100)*0.55);
    colormap(ax, [1 1 1; 0.85 0.25 0.25]);
    set(ax, 'YDir','normal', 'Layer','top');

    hBody = plot(body_world(:,1),...
        body_world(:,2),...
        'k','LineWidth',2);

    hWheelFL = plot(wheelFL(:,1),...
        wheelFL(:,2),...
        'r','LineWidth',2);

    hWheelFR = plot(wheelFR(:,1),...
        wheelFR(:,2),...
        'r','LineWidth',2);

    hWheelRL = plot(wheelRL(:,1),...
        wheelRL(:,2),...
        'b','LineWidth',2);

    hWheelRR = plot(wheelRR(:,1),...
        wheelRR(:,2),...
        'b','LineWidth',2);

    TrajX = x;
    TrajY = y;

   hTrajectory = plot(TrajX, TrajY, 'g', 'LineWidth', 3);
   hRefTraj    = plot(x_ref, y_ref, 'b', 'LineWidth', 1);

else

    set(hBody,...
        'XData',body_world(:,1),...
        'YData',body_world(:,2));

    set(hWheelFL,...
        'XData',wheelFL(:,1),...
        'YData',wheelFL(:,2));

    set(hWheelFR,...
        'XData',wheelFR(:,1),...
        'YData',wheelFR(:,2));

    set(hWheelRL,...
        'XData',wheelRL(:,1),...
        'YData',wheelRL(:,2));

    set(hWheelRR,...
        'XData',wheelRR(:,1),...
        'YData',wheelRR(:,2));

    TrajX(end+1) = x;
    TrajY(end+1) = y;

 
    set(hTrajectory,...
        'XData',TrajX,...
        'YData',TrajY);

    set(hRefTraj,...
        'XData',x_ref,...
        'YData',y_ref);

end

   xlim(ax, [-16 16])
   ylim(ax, [-14 14])

% xlim([-20 20])
% ylim([-20 20])

drawnow limitrate


end

== matlab function ATOM_simple_planning_simulator/Plot vehicle1/Plot vehicle Front reference frame ==
  settings: updateMethod=DISCRETE
  data: kinematic input Bus: KinematicStateBus; steer_front input double; steer_rear input double; veh input; traj input
function plotVehicleFront(kinematic, steer_front, steer_rear, veh, traj)

%% Vehicle parameters

L  = veh(3);
track = veh(4);

front_overhang = veh(5);
rear_overhang  = veh(6);
left_overhang = veh(7);
right_overhang = veh(8);

vehicle_length  = L + front_overhang + rear_overhang;
vehicle_width = track + left_overhang + right_overhang;

wheel_width = veh(2);
wheel_radius = veh(1);

%% Reference trajectory

x_ref = traj.pose.position.x;
y_ref = traj.pose.position.y;

yaw_ref = zeros(length(x_ref),1);


for i=1:length(x_ref)

    yaw_ref(i)=2*atan2(...
        traj.pose.orientation.qz(i),...
        traj.pose.orientation.qw(i));
end


%% Current kinematic state

x = kinematic.pose.position.x;
y = kinematic.pose.position.y;

qz = kinematic.pose.orientation.z;
qw = kinematic.pose.orientation.w;

yaw = 2*atan2(qz,qw);

vx = kinematic.twist.linear.x;

steer_front = steer_front;
steer_rear = steer_rear;

%% Position and orientation vehicle body

vehicle_body = [front_overhang vehicle_width/2;
                front_overhang -vehicle_width/2;
                -L-rear_overhang -vehicle_width/2;
                -L-rear_overhang vehicle_width/2;
                front_overhang vehicle_width/2];

R_body = [ cos(yaw) -sin(yaw)
    sin(yaw)  cos(yaw) ];

body_world = (R_body*vehicle_body')';

body_world(:,1)=body_world(:,1)+x;
body_world(:,2)=body_world(:,2)+y;


%% Position and orientation wheels

wheel_body = [wheel_radius  wheel_width/2
                wheel_radius -wheel_width/2
                -wheel_radius -wheel_width/2
                -wheel_radius  wheel_width/2
                wheel_radius  wheel_width/2];

FL = [0  track/2];
FR = [0 -track/2];
RL = [-L  track/2];
RR = [-L -track/2];

centers = [FL;
    FR;
    RL;
    RR];

centers = (R_body*centers')';

centers(:,1) = centers(:,1)+x;
centers(:,2) = centers(:,2)+y;

wheelFL = transformWheel(centers(1,:),steer_front,yaw,wheel_body);
wheelFR = transformWheel(centers(2,:),steer_front,yaw,wheel_body);
wheelRL = transformWheel(centers(3,:),steer_rear,yaw,wheel_body);
wheelRR = transformWheel(centers(4,:),steer_rear,yaw,wheel_body);



persistent hFig
persistent ax
persistent hBody
persistent hWheelFL
persistent hWheelFR
persistent hWheelRL
persistent hWheelRR
persistent hTrajectory
persistent TrajX
persistent TrajY
persistent hRefTraj 
persistent hArrow


if isempty(hBody)
    hFig = figure(13);
    clf

    ax = axes(hFig);

    hold(ax,'on')
    axis(ax,'equal')
    grid(ax,'on')


    xlabel(ax,'x [m]')
    ylabel(ax,'y [m]')

    hBody = plot(body_world(:,1),...
        body_world(:,2),...
        'k','LineWidth',2);

    hWheelFL = plot(wheelFL(:,1),...
        wheelFL(:,2),...
        'r','LineWidth',2);

    hWheelFR = plot(wheelFR(:,1),...
        wheelFR(:,2),...
        'r','LineWidth',2);

    hWheelRL = plot(wheelRL(:,1),...
        wheelRL(:,2),...
        'b','LineWidth',2);

    hWheelRR = plot(wheelRR(:,1),...
        wheelRR(:,2),...
        'b','LineWidth',2);

    TrajX = x;
    TrajY = y;

    hTrajectory = plot(TrajX,...
                       TrajY,...
                       'g','LineWidth',1);

    hRefTraj=plot(x_ref,y_ref,'b','LineWidth',2);

    step=5;

    hArrow=quiver(...
        x_ref(1:step:end),...
        y_ref(1:step:end),...
        cos(yaw_ref(1:step:end)),...
        sin(yaw_ref(1:step:end)),...
        0.5,...
        'r');

else

    set(hBody,...
        'XData',body_world(:,1),...
        'YData',body_world(:,2));

    set(hWheelFL,...
        'XData',wheelFL(:,1),...
        'YData',wheelFL(:,2));

    set(hWheelFR,...
        'XData',wheelFR(:,1),...
        'YData',wheelFR(:,2));

    set(hWheelRL,...
        'XData',wheelRL(:,1),...
        'YData',wheelRL(:,2));

    set(hWheelRR,...
        'XData',wheelRR(:,1),...
        'YData',wheelRR(:,2));

    TrajX(end+1) = x;
    TrajY(end+1) = y;

 
    set(hTrajectory,...
        'XData',TrajX,...
        'YData',TrajY);

    set(hRefTraj,...
        'XData',x_ref,...
        'YData',y_ref);

    

end

margin = 12;
xlim(ax, [x-margin x+margin])
ylim(ax, [y-margin y+margin])

% xlim([-20 20])
% ylim([-20 20])

drawnow limitrate


end

== matlab function ATOM_simple_planning_simulator/Plot vehicle1/RearToFrontOdometry ==
  data: rear_pose input Bus: KinematicStateBus; front_pose output Bus: KinematicStateBus; wheel_base input
function front_pose = RearToFrontOdometry( ...
    rear_pose,...
    wheel_base)


front_pose = rear_pose;


qx = rear_pose.pose.orientation.x;
qy = rear_pose.pose.orientation.y;
qz = rear_pose.pose.orientation.z;
qw = rear_pose.pose.orientation.w;


yaw = QuaternionToYaw(qx,qy,qz,qw);



front_pose.pose.position.x = ...
    rear_pose.pose.position.x + ...
    wheel_base*cos(yaw);


front_pose.pose.position.y = ...
    rear_pose.pose.position.y + ...
    wheel_base*sin(yaw);


front_pose.pose.position.z = ...
    rear_pose.pose.position.z;



% orientation unchanged

front_pose.pose.orientation = ...
    rear_pose.pose.orientation;


% Linear velocity referred to front axle

front_pose.twist.linear.x = rear_pose.twist.linear.x ...
    - rear_pose.twist.angular.z ...
    * wheel_base*sin(yaw);


front_pose.twist.linear.y = rear_pose.twist.linear.y ...
    + rear_pose.twist.angular.z ...
    * wheel_base*cos(yaw);


front_pose.twist.linear.z = rear_pose.twist.linear.z;


end

== matlab function ATOM_simple_planning_simulator/Plot demanded trajectory ==
  data: traj input
function plotTrajectory(traj)

persistent hTraj hArrow


x = traj.pose.position.x;
y = traj.pose.position.y;

yaw = zeros(length(x),1);


for i=1:length(x)

    yaw(i)=2*atan2(...
        traj.pose.orientation.qz(i),...
        traj.pose.orientation.qw(i));

end


if isempty(hTraj)

    figure(2)
    clf
    hold on
    grid on
    axis equal

    hTraj=plot(x,y,'b','LineWidth',2);


    step=5;

    hArrow=quiver(...
        x(1:step:end),...
        y(1:step:end),...
        cos(yaw(1:step:end)),...
        sin(yaw(1:step:end)),...
        0.5,...
        'r');

else

    set(hTraj,...
        'XData',x,...
        'YData',y);

end


drawnow limitrate

end
